simulink model "otherNoiseStudies"  (R2017b)
settings: Solver=VariableStepAuto  StartTime=0.0  StopTime=time(end)  RelTol=1e-3
undefined symbols (not defined in the file): ST
settings Model: Creator=CC  LastModifiedBy=CC

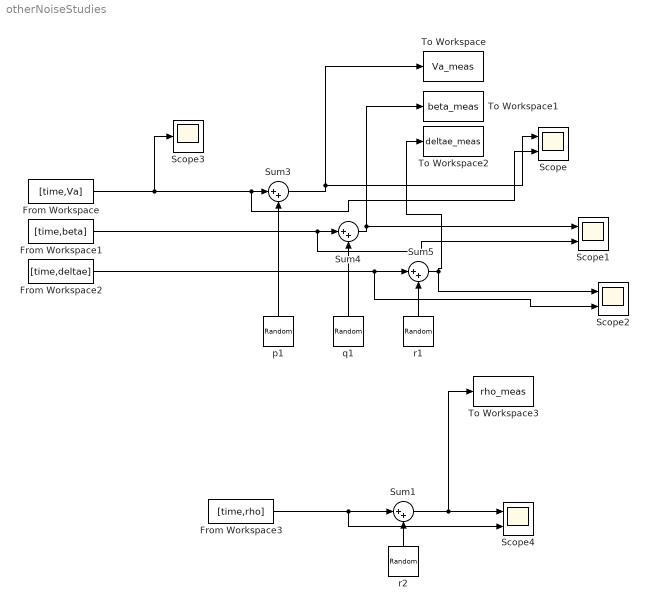
== system otherNoiseStudies ==
  From Workspace : FromWorkspace  VariableName=[time,Va]  SampleTime=0
  From Workspace1 : FromWorkspace  VariableName=[time,beta]  SampleTime=0
  From Workspace2 : FromWorkspace  VariableName=[time,deltae]  SampleTime=0
  From Workspace3 : FromWorkspace  VariableName=[time,rho]  SampleTime=0
  Scope{,1..2,4} (4 alike) : Scope  NumInputPorts=2
  Scope3 : Scope
  Sum{1,3..5} (4 alike) : Sum  Inputs=|++
  To Workspace : ToWorkspace  VariableName=Va_meas  SampleTime=-1
  To Workspace1 : ToWorkspace  VariableName=beta_meas  SampleTime=-1
  To Workspace2 : ToWorkspace  VariableName=deltae_meas  SampleTime=-1
  To Workspace3 : ToWorkspace  VariableName=rho_meas  SampleTime=-1
  p1 : RandomNumber  Variance=0.01  SampleTime=ST
  q1 : RandomNumber  Variance=0.001  SampleTime=ST
  r1 : RandomNumber  Variance=0.001  SampleTime=ST
  r2 : RandomNumber  Variance=0.00001  SampleTime=ST
  wires:
  Sum4/1 -> To Workspace1/1, Scope1/1
  Sum3/1 -> To Workspace/1, Scope/1
  Sum5/1 -> To Workspace2/1, Scope2/1
  p1/1 -> Sum3/2
  From Workspace2/1 -> Scope2/2, Sum5/1
  q1/1 -> Sum4/2
  From Workspace1/1 -> Scope1/2, Sum4/1
  From Workspace/1 -> Scope3/1, Scope/2, Sum3/1
  r1/1 -> Sum5/2
  From Workspace3/1 -> Scope4/2, Sum1/1
  r2/1 -> Sum1/2
  Sum1/1 -> To Workspace3/1, Scope4/1
